simulink model "latest_coil"  (R2021b)
settings: Solver=FixedStepAuto  StartTime=-18e-3  StopTime=50e-3  FixedStep=1e-4  RelTol=1e-3
undefined symbols (not defined in the file): X, Y, Z
libraries: sm_lib x28, nesl_utility x9
(part 5 of 5)

== matlab function latest_coil/MATLAB Function2 ==
  data: Ff_x output; Fext_x input; vx input
function Ff_x = friction(Fext_x,vx)
Coeff_of_Fric = 0.432;
g = 9.8;
mass_of_bot = 9.17345e-05;

% if  Fext_x < 0 && vx >= 0 %When force is in negative direction and velocity is in positive direction (impossible case) (Removing this case implies object doesn't move)
%     Ff_x = 0;
% elseif  Fext_x > 0 && vx <= 0 %When force is in positivedirection and velocity is in positive direction (impossible case)
%     Ff_x = 0;
% elseif  vx < 0 %When velocity is in negative direction friction is positive (Object is moving)
%     Ff_x = Coeff_of_Fric*mass_of_bot*g;
% elseif  vx > 0 %When velocity is in positive direction friction is negative (Object is moving)
%     Ff_x = -Coeff_of_Fric*mass_of_bot*g;
% elseif (abs(Fext_x) >= Coeff_of_Fric*mass_of_bot*g  &&  vx < 0 ) || (abs(Fext_x) >= Coeff_of_Fric*mass_of_bot*g && vx > 0) %When applied force greater than couloumb friction and 
%                                                                                                                        % moves is positive or negative direction, then Couloumb friction opposes that motion
%     Ff_x = -Coeff_of_Fric*mass_of_bot*g*sign(Fext_x);
% 
% elseif (abs(Fext_x) < Coeff_of_Fric*mass_of_bot*g && Fext_x~= 0) %When applied force less than Coloumb Friction but not equal to zero, Friction force is applied force
%     Ff_x = -Fext_x;
% else %When applied force is zero or when object not moving
%     Ff_x = -Fext_x;
% end

if abs(vx)<0.01
    if abs(Fext_x)>Coeff_of_Fric*mass_of_bot*g
        Ff_x=-Coeff_of_Fric*mass_of_bot*g*sign(Fext_x);
    else
        Ff_x=-Fext_x-vx;
    end
else
    Ff_x=-Coeff_of_Fric*mass_of_bot*g*sign(vx);
end

== matlab function latest_coil/Inner Coil/Coil 1/MATLAB Function4 ==
  data: Hx_xp input; Hy_xp input; Hz_xp input; Hx output; Hx_xn input; Hy_xn input; Hy output; Hz output; Hz_xn input; Hx_yp input; Hy_yp input; Hz_yp input; Hx_yn input; Hy_yn input; Hz_yn input
function [Hx, Hy, Hz] = field_sum(Hx_xp, Hy_xp, Hz_xp, Hx_xn, Hy_xn, Hz_xn, Hx_yp, Hy_yp, Hz_yp, Hx_yn, Hy_yn, Hz_yn)
Hx = Hx_xp + Hx_xn + Hx_yp + Hx_yn;
Hy = Hy_xp + Hy_xn + Hy_yp + Hy_yn;
Hz = Hz_xp + Hz_xn + Hz_yp + Hz_yn;
end

== matlab function latest_coil/Inner Coil/Coil 2/FIELD_X ==
  data: X input; Hx_xp output; Y input; Z input; I input; Hy_xp output; Hz_xp output; Hx_xn output; Hy_xn output; Hz_xn output; dBy_dx output; dBy_dy output; dBy_dz output; dBz_dx output; dBz_dy output; dBz_dz output
function [Hx_xp, Hy_xp, Hz_xp, Hx_xn, Hy_xn, Hz_xn,dBy_dx ,dBy_dy, dBy_dz, dBz_dx ,dBz_dy, dBz_dz] = field_x(X, Y, Z, I)
n = 2;
gx = 1.075e-3;
gz = 0;
m0 = 4*pi*1e-7;
k = 0.4e-3;
xp1 = -0.8e-3 - (n-1)*k;
xp2 = 0.8e-3 + (n-1)*k;
a_yp = gx; 
a_zp = gz;
k_p = 1./(4*pi*((a_yp-Y).^2+(a_zp-Z).^2));
kxp = (xp2-X)./((xp2-X).^2+(a_yp-Y).^2+(a_zp-Z).^2).^0.5;
k_2xp = (xp1-X)./((xp1-X).^2+(a_yp-Y).^2+(a_zp-Z).^2).^0.5;

Hx_xp = zeros(size(X,1),size(Y,1),size(Z,1));
Hy_xp = (-(a_zp-Z).*k_p.*(kxp - k_2xp))*I*m0;
Hz_xp = (-(a_yp-Y).*k_p.*(kxp - k_2xp))*I*m0;

a_yn = -gx;
xn1 = -1e-3 - (n-1)*k;
xn2 = 1e-3 + (n-1)*k;
k_n = 1./(4*pi*((a_yn-Y).^2+(a_zp-Z).^2));
kxn = (xn2-X)./((xn2-X).^2+(a_yn-Y).^2+(a_zp-Z).^2).^0.5;
k_2xn = (xn1-X)./((xn1-X).^2+(a_yn-Y).^2+(a_zp-Z).^2).^0.5;

Hx_xn = zeros(size(X,1),size(Y,1),size(Z,1));
Hy_xn = ((a_zp-Z).*k_n.*(kxn - k_2xn))*I*m0;
Hz_xn = ((a_yn-Y).*k_n.*(kxn - k_2xn))*I*m0;

dByn_dx = (I*Z*m0*(1/((Y - a_yn)^2 + (Z - a_zp)^2 + (X - xn1)^2)^(1/2) - 1/((Y - a_yn)^2 + (Z - a_zp)^2 + (X - xn2)^2)^(1/2) - ((X - xn1)*(2*X - 2*xn1))/(2*((Y - a_yn)^2 + (Z - a_zp)^2 + (X - xn1)^2)^(3/2)) + ((X - xn2)*(2*X - 2*xn2))/(2*((Y - a_yn)^2 + (Z - a_zp)^2 + (X - xn2)^2)^(3/2))))/(4*pi*((Y - a_yn)^2 + (Z - a_zp)^2));
dByp_dx = -(I*Z*m0*(1/((Y - a_yp)^2 + (Z - a_zp)^2 + (X - xp1)^2)^(1/2) - 1/((Y - a_yp)^2 + (Z - a_zp)^2 + (X - xp2)^2)^(1/2) - ((X - xp1)*(2*X - 2*xp1))/(2*((Y - a_yp)^2 + (Z - a_zp)^2 + (X - xp1)^2)^(3/2)) + ((X - xp2)*(2*X - 2*xp2))/(2*((Y - a_yp)^2 + (Z - a_zp)^2 + (X - xp2)^2)^(3/2))))/(4*pi*((Y - a_yp)^2 + (Z - a_zp)^2));
dBy_dx = dByp_dx + dByn_dx;

dByp_dy = (I*Z*m0*(((X - xp1)*(2*Y - 2*a_yp))/(2*((Y - a_yp)^2 + (Z - a_zp)^2 + (X - xp1)^2)^(3/2)) - ((X - xp2)*(2*Y - 2*a_yp))/(2*((Y - a_yp)^2 + (Z - a_zp)^2 + (X - xp2)^2)^(3/2))))/(4*pi*((Y - a_yp)^2 + (Z - a_zp)^2)) + (I*Z*m0*(2*Y - 2*a_yp)*((X - xp1)/((Y - a_yp)^2 + (Z - a_zp)^2 + (X - xp1)^2)^(1/2) - (X - xp2)/((Y - a_yp)^2 + (Z - a_zp)^2 + (X - xp2)^2)^(1/2)))/(4*pi*((Y - a_yp)^2 + (Z - a_zp)^2)^2);
dByn_dy = - (I*Z*m0*(((X - xn1)*(2*Y - 2*a_yn))/(2*((Y - a_yn)^2 + (Z - a_zp)^2 + (X - xn1)^2)^(3/2)) - ((X - xn2)*(2*Y - 2*a_yn))/(2*((Y - a_yn)^2 + (Z - a_zp)^2 + (X - xn2)^2)^(3/2))))/(4*pi*((Y - a_yn)^2 + (Z - a_zp)^2)) - (I*Z*m0*(2*Y - 2*a_yn)*((X - xn1)/((Y - a_yn)^2 + (Z - a_zp)^2 + (X - xn1)^2)^(1/2) - (X - xn2)/((Y - a_yn)^2 + (Z - a_zp)^2 + (X - xn2)^2)^(1/2)))/(4*pi*((Y - a_yn)^2 + (Z - a_zp)^2)^2);
dBy_dy = dByp_dy + dByn_dy;

dByp_dz = (I*Z*m0*(((X - xp1)*(2*Z - 2*a_zp))/(2*((Y - a_yp)^2 + (Z - a_zp)^2 + (X - xp1)^2)^(3/2)) - ((X - xp2)*(2*Z - 2*a_zp))/(2*((Y - a_yp)^2 + (Z - a_zp)^2 + (X - xp2)^2)^(3/2))))/(4*pi*((Y - a_yp)^2 + (Z - a_zp)^2)) - (I*m0*((X - xp1)/((Y - a_yp)^2 + (Z - a_zp)^2 + (X - xp1)^2)^(1/2) - (X - xp2)/((Y - a_yp)^2 + (Z - a_zp)^2 + (X - xp2)^2)^(1/2)))/(4*pi*((Y - a_yp)^2 + (Z - a_zp)^2)) + (I*Z*m0*(2*Z - 2*a_zp)*((X - xp1)/((Y - a_yp)^2 + (Z - a_zp)^2 + (X - xp1)^2)^(1/2) - (X - xp2)/((Y - a_yp)^2 + (Z - a_zp)^2 + (X - xp2)^2)^(1/2)))/(4*pi*((Y - a_yp)^2 + (Z - a_zp)^2)^2);
dByn_dz = (I*m0*((X - xn1)/((Y - a_yn)^2 + (Z - a_zp)^2 + (X - xn1)^2)^(1/2) - (X - xn2)/((Y - a_yn)^2 + (Z - a_zp)^2 + (X - xn2)^2)^(1/2)))/(4*pi*((Y - a_yn)^2 + (Z - a_zp)^2)) - (I*Z*m0*(((X - xn1)*(2*Z - 2*a_zp))/(2*((Y - a_yn)^2 + (Z - a_zp)^2 + (X - xn1)^2)^(3/2)) - ((X - xn2)*(2*Z - 2*a_zp))/(2*((Y - a_yn)^2 + (Z - a_zp)^2 + (X - xn2)^2)^(3/2))))/(4*pi*((Y - a_yn)^2 + (Z - a_zp)^2)) - (I*Z*m0*(2*Z - 2*a_zp)*((X - xn1)/((Y - a_yn)^2 + (Z - a_zp)^2 + (X - xn1)^2)^(1/2) - (X - xn2)/((Y - a_yn)^2 + (Z - a_zp)^2 + (X - xn2)^2)^(1/2)))/(4*pi*((Y - a_yn)^2 + (Z - a_zp)^2)^2);
dBy_dz = dByp_dz + dByn_dz;

dBzp_dx = (I*m0*(Y - a_yp)*(1/((Y - a_yp)^2 + (Z - a_zp)^2 + (X - xp1)^2)^(1/2) - 1/((Y - a_yp)^2 + (Z - a_zp)^2 + (X - xp2)^2)^(1/2) - ((X - xp1)*(2*X - 2*xp1))/(2*((Y - a_yp)^2 + (Z - a_zp)^2 + (X - xp1)^2)^(3/2)) + ((X - xp2)*(2*X - 2*xp2))/(2*((Y - a_yp)^2 + (Z - a_zp)^2 + (X - xp2)^2)^(3/2))))/(4*pi*(Z^2 + (Y - a_yp)^2));
dBzn_dx = -(I*m0*(Y - a_yn)*(1/((Y - a_yn)^2 + (Z - a_zp)^2 + (X - xn1)^2)^(1/2) - 1/((Y - a_yn)^2 + (Z - a_zp)^2 + (X - xn2)^2)^(1/2) - ((X - xn1)*(2*X - 2*xn1))/(2*((Y - a_yn)^2 + (Z - a_zp)^2 + (X - xn1)^2)^(3/2)) + ((X - xn2)*(2*X - 2*xn2))/(2*((Y - a_yn)^2 + (Z - a_zp)^2 + (X - xn2)^2)^(3/2))))/(4*pi*(Z^2 + (Y - a_yn)^2));
dBz_dx = dBzp_dx + dBzn_dx;

dBzn_dy = (I*m0*(Y - a_yn)*(((X - xn1)*(2*Y - 2*a_yn))/(2*((Y - a_yn)^2 + (Z - a_zp)^2 + (X - xn1)^2)^(3/2)) - ((X - xn2)*(2*Y - 2*a_yn))/(2*((Y - a_yn)^2 + (Z - a_zp)^2 + (X - xn2)^2)^(3/2))))/(4*pi*(Z^2 + (Y - a_yn)^2)) - (I*m0*((X - xn1)/((Y - a_yn)^2 + (Z - a_zp)^2 + (X - xn1)^2)^(1/2) - (X - xn2)/((Y - a_yn)^2 + (Z - a_zp)^2 + (X - xn2)^2)^(1/2)))/(4*pi*(Z^2 + (Y - a_yn)^2)) + (I*m0*(Y - a_yn)*(2*Y - 2*a_yn)*((X - xn1)/((Y - a_yn)^2 + (Z - a_zp)^2 + (X - xn1)^2)^(1/2) - (X - xn2)/((Y - a_yn)^2 + (Z - a_zp)^2 + (X - xn2)^2)^(1/2)))/(4*pi*(Z^2 + (Y - a_yn)^2)^2);
dBzp_dy = (I*m0*((X - xp1)/((Y - a_yp)^2 + (Z - a_zp)^2 + (X - xp1)^2)^(1/2) - (X - xp2)/((Y - a_yp)^2 + (Z - a_zp)^2 + (X - xp2)^2)^(1/2)))/(4*pi*(Z^2 + (Y - a_yp)^2)) - (I*m0*(Y - a_yp)*(((X - xp1)*(2*Y - 2*a_yp))/(2*((Y - a_yp)^2 + (Z - a_zp)^2 + (X - xp1)^2)^(3/2)) - ((X - xp2)*(2*Y - 2*a_yp))/(2*((Y - a_yp)^2 + (Z - a_zp)^2 + (X - xp2)^2)^(3/2))))/(4*pi*(Z^2 + (Y - a_yp)^2)) - (I*m0*(Y - a_yp)*(2*Y - 2*a_yp)*((X - xp1)/((Y - a_yp)^2 + (Z - a_zp)^2 + (X - xp1)^2)^(1/2) - (X - xp2)/((Y - a_yp)^2 + (Z - a_zp)^2 + (X - xp2)^2)^(1/2)))/(4*pi*(Z^2 + (Y - a_yp)^2)^2);
dBz_dy = dBzn_dy + dBzp_dy;

dBzn_dz = (I*m0*(Y - a_yn)*(((X - xn1)*(2*Z - 2*a_zp))/(2*((Y - a_yn)^2 + (Z - a_zp)^2 + (X - xn1)^2)^(3/2)) - ((X - xn2)*(2*Z - 2*a_zp))/(2*((Y - a_yn)^2 + (Z - a_zp)^2 + (X - xn2)^2)^(3/2))))/(4*pi*(Z^2 + (Y - a_yn)^2)) + (I*Z*m0*(Y - a_yn)*((X - xn1)/((Y - a_yn)^2 + (Z - a_zp)^2 + (X - xn1)^2)^(1/2) - (X - xn2)/((Y - a_yn)^2 + (Z - a_zp)^2 + (X - xn2)^2)^(1/2)))/(2*pi*(Z^2 + (Y - a_yn)^2)^2);
dBzp_dz = - (I*m0*(Y - a_yp)*(((X - xp1)*(2*Z - 2*a_zp))/(2*((Y - a_yp)^2 + (Z - a_zp)^2 + (X - xp1)^2)^(3/2)) - ((X - xp2)*(2*Z - 2*a_zp))/(2*((Y - a_yp)^2 + (Z - a_zp)^2 + (X - xp2)^2)^(3/2))))/(4*pi*(Z^2 + (Y - a_yp)^2)) - (I*Z*m0*(Y - a_yp)*((X - xp1)/((Y - a_yp)^2 + (Z - a_zp)^2 + (X - xp1)^2)^(1/2) - (X - xp2)/((Y - a_yp)^2 + (Z - a_zp)^2 + (X - xp2)^2)^(1/2)))/(2*pi*(Z^2 + (Y - a_yp)^2)^2);
dBz_dz = dBzn_dz + dBzp_dz;
end
